simulink library "PosControl"  (R2024a)
settings: Solver=VariableStepAuto  StartTime=0.0  StopTime=10.0  RelTol=1e-3
undefined symbols (not defined in the file): AltHold_Freq, PSC_ACCZ_D, PSC_ACCZ_I, PSC_ACCZ_P, PSC_POSZ_P, PSC_VELZ_D, PSC_VELZ_I, PSC_VELZ_P, THR_CLIMB_MAX, THR_SINK_MAX
libraries: ArdupilotFunctions x2
settings Model: Creator=igmso  LastModifiedBy=igmso

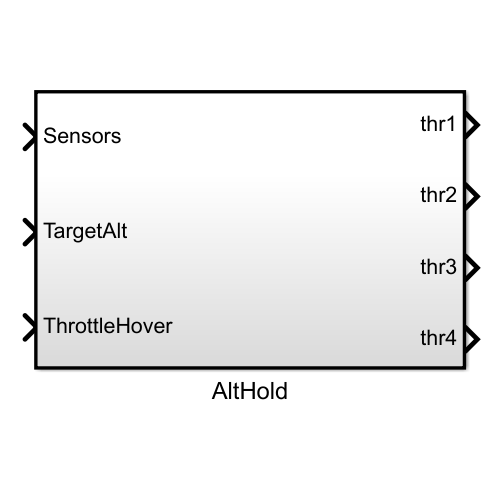
[thumbnail: Simulink's stored preview of the top-level diagram]
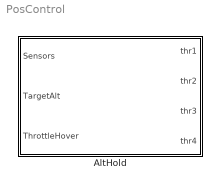
== system PosControl ==
  AltHold : Subsystem  TreatAsAtomicUnit=on

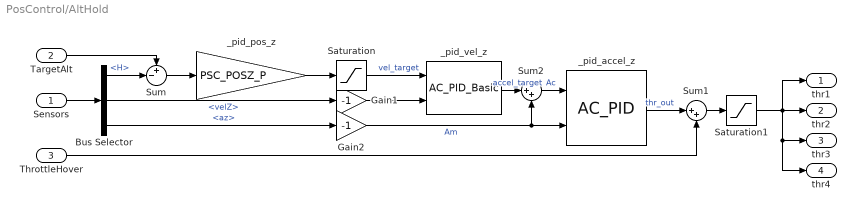
== system PosControl/AltHold ==
  Sensors : Inport  SampleTime=1/AltHold_Freq
  TargetAlt : Inport  Port=2  SampleTime=1/AltHold_Freq
  ThrottleHover : Inport  Port=3  SampleTime=1/AltHold_Freq
  Bus Selector : BusSelector  OutputSignals=H,velZ,az
  Gain1 : Gain  Gain=-1
  Gain2 : Gain  Gain=-1
  Saturation : Saturate  UpperLimit=THR_CLIMB_MAX  LowerLimit=-THR_SINK_MAX
  Saturation1 : Saturate  UpperLimit=1  LowerLimit=0
  Sum : Sum  Inputs=+-|
  Sum1 : Sum  Inputs=|++
  Sum2 : Sum  Inputs=|++
  _pid_accel_z : ArdupilotFunctions/AC_PID  P=PSC_ACCZ_P  I=PSC_ACCZ_I  D=PSC_ACCZ_D  FF=PSC_ACCZ_FF  D_FF=PSC_ACCZ_D_FF  FLTD=PSC_ACCZ_FLTD  FLTE=PSC_ACCZ_FLTE  FLTT=PSC_ACCZ_FLTT  IMAX=PSC_ACCZ_IMAX
  _pid_pos_z : Gain  Gain=PSC_POSZ_P
  _pid_vel_z : ArdupilotFunctions/AC_PID_Basic  P=PSC_VELZ_P  I=PSC_VELZ_I  D=PSC_VELZ_D  FF=PSC_VELZ_FF  FLTD=PSC_VELZ_FLTD  FLTE=PSC_VELZ_FLTE  IMAX=PSC_VELZ_IMAX
  thr1 : Outport  SampleTime=1/AltHold_Freq
  thr2 : Outport  Port=2  SampleTime=1/AltHold_Freq
  thr3 : Outport  Port=3  SampleTime=1/AltHold_Freq
  thr4 : Outport  Port=4  SampleTime=1/AltHold_Freq
  wires:
  TargetAlt/1 -> Sum/1
  Saturation/1 -> _pid_vel_z/1  "vel_target"
  Sum2/1 -> _pid_accel_z/1  "Ac"
  _pid_vel_z/1 -> Sum2/1  "accel_target"
  Gain2/1 -> _pid_accel_z/2, Sum2/2  "Am"
  Saturation1/1 -> thr1/1, thr4/1, thr3/1, thr2/1
  ThrottleHover/1 -> Sum1/2
  _pid_accel_z/1 -> Sum1/1  "thr_out"
  Bus Selector/3 -> Gain2/1  "<az>"
  Bus Selector/2 -> Gain1/1  "<velZ>"
  _pid_pos_z/1 -> Saturation/1
  Sum/1 -> _pid_pos_z/1
  Bus Selector/1 -> Sum/2  "<H>"
  Sensors/1 -> Bus Selector/1
  Sum1/1 -> Saturation1/1
  Gain1/1 -> _pid_vel_z/2
